simulink model "eq_2_9_model_e"  (R2025a)
settings: Solver=VariableStepAuto  StartTime=0.0  StopTime=500  RelTol=1e-3
values from neighbouring files (symbols this model uses):
  Ka = 1    [c29.m]    (also in d29.m; e29.m)
  Kc = 110    [c29.m]    (also in d29.m; e29.m)
  Kf = 2.5    [c29.m]    (also in d29.m; e29.m)
  Ki = 15    [c29.m]    (also in d29.m = 90; e29.m)
  Kp = 500    [c29.m]    (also in d29.m; e29.m)
  m = 1500    [c29.m]    (also in d29.m; e29.m)
  vd = 30    [c29.m]    (also in d29.m; e29.m)
  x10 = 0    [c29.m]    (also in d29.m; e29.m)
  x20 = 0    [c29.m]    (also in d29.m; e29.m)
settings Model: Creator=Nenad  LastModifiedBy=Korisnik

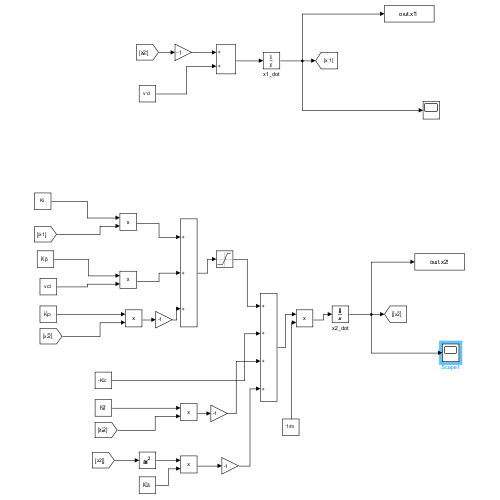
[thumbnail: Simulink's stored preview of the top-level diagram]
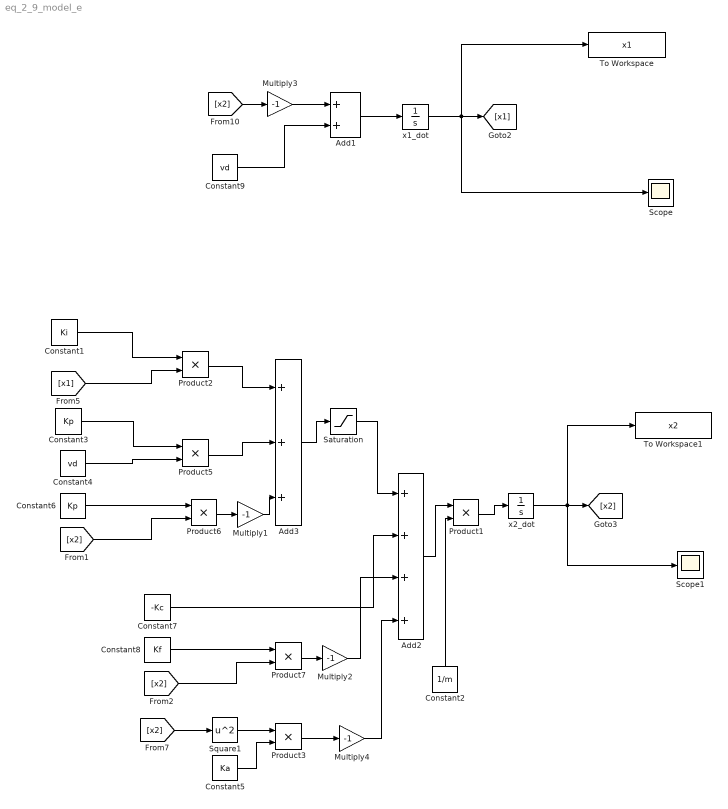
== system eq_2_9_model_e ==
  Add1 : Sum  Inputs=2
  Add2 : Sum  Inputs=4
  Add3 : Sum  Inputs=3
  Constant1 : Constant  Value=Ki
  Constant2 : Constant  Value=1/m
  Constant3 : Constant  Value=Kp
  Constant4 : Constant  Value=vd
  Constant5 : Constant  Value=Ka
  Constant6 : Constant  Value=Kp
  Constant7 : Constant  Value=-Kc
  Constant8 : Constant  Value=Kf
  Constant9 : Constant  Value=vd
  Multiply{1..4} (4 alike) : Gain  Gain=-1
  Product{1..3,5..7} (6 alike) : Product
  Saturation : Saturate  UpperLimit=1800  LowerLimit=0
  Scope : Scope
      settings: ActiveDisplayYMinimum=-82.308545417818351  ActiveDisplayYMaximum=343.77272035951023
  Scope1 : Scope
      settings: ActiveDisplayYMinimum=-327.85412792035441  ActiveDisplayYMaximum=340.5603393766782
  Square1 : Math  Operator=square
  To Workspace : ToWorkspace  VariableName=x1  SaveFormat=Timeseries  SampleTime=-1
  To Workspace1 : ToWorkspace  VariableName=x2  SaveFormat=Timeseries  SampleTime=-1
  x1_dot : Integrator  InitialCondition=x10
  x2_dot : Integrator  InitialCondition=x20
  wires:
  x1_dot/1 -> Scope/1, To Workspace/1, [x1]
  x2_dot/1 -> Scope1/1, To Workspace1/1, [x2]
  [x1] -> Product2/2
  Constant1/1 -> Product2/1
  Add2/1 -> Product1/1
  Product1/1 -> x2_dot/1
  Constant2/1 -> Product1/2
  [x2] -> Square1/1
  Product3/1 -> Multiply4/1
  Constant5/1 -> Product3/2
  Square1/1 -> Product3/1
  Constant3/1 -> Product5/1
  Constant4/1 -> Product5/2
  Constant6/1 -> Product6/1
  [x2] -> Product6/2
  Product6/1 -> Multiply1/1
  [x2] -> Product7/2
  Constant8/1 -> Product7/1
  Product7/1 -> Multiply2/1
  [x2] -> Multiply3/1
  Constant9/1 -> Add1/2
  Multiply3/1 -> Add1/1
  Add1/1 -> x1_dot/1
  Constant7/1 -> Add2/2
  Multiply2/1 -> Add2/3
  Multiply4/1 -> Add2/4
  Product2/1 -> Add3/1
  Product5/1 -> Add3/2
  Multiply1/1 -> Add3/3
  Add3/1 -> Saturation/1
  Saturation/1 -> Add2/1
